simulink model "untitled"  (R2022b)
settings: Solver=VariableStepAuto  StartTime=0.0  StopTime=10.0  RelTol=1e-3
settings Model: Creator=Dell  LastModifiedBy=Dell

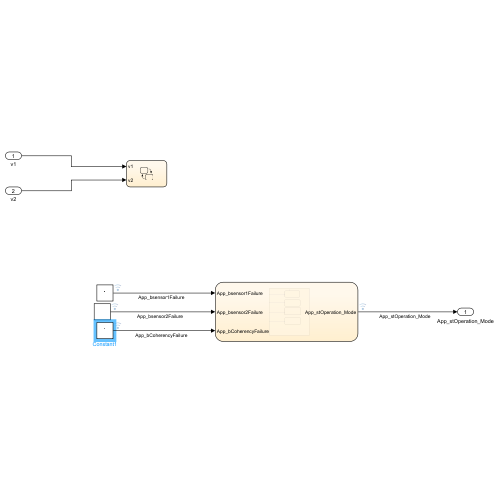
[thumbnail: Simulink's stored preview of the top-level diagram]
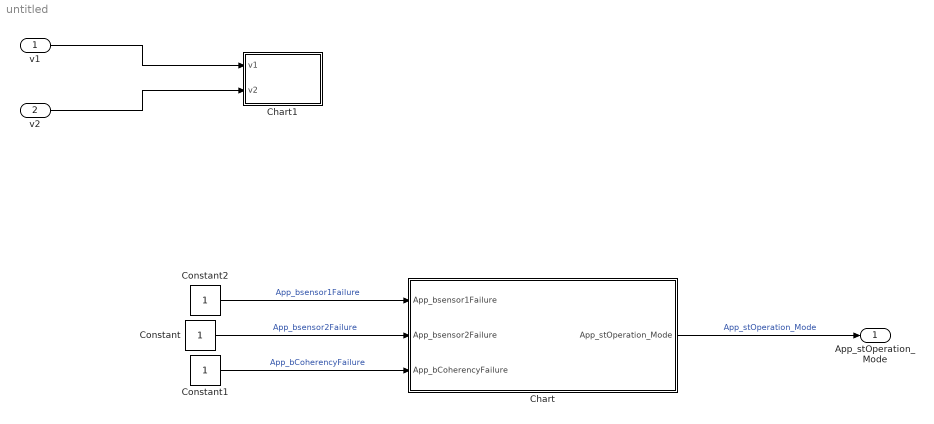
== system untitled ==
  v1 : Inport
  v2 : Inport  Port=2
  Chart : Stateflow chart  TreatAsAtomicUnit=on
  Chart1 : Stateflow chart  TreatAsAtomicUnit=on
      settings: PortSchema="{\"entries\":[{\"content\":{\"sides\":[{\"content\":{\"connectorIds\":[\"In2\",\"In1\"]},\"type\":\"ConnectorPlacement.EquallySpacedRectSide\",\"uuid\":\"969f0c33-844b-45d6-9c47-d424376eedef\"},{\"content\":{\"connectorIds\":[],\"side\":\"RIGHT\"},\"type\":\"ConnectorPlacement.EquallySpacedRectSide\",\"uuid\":\"6fc1ba59-4f2d-4ccb-a718-6a4f6694da1f\"},{\"content\":{\"connectorIds\":[],\"side\":\"TOP\"},\"type\":\"ConnectorPlacement.EquallySpacedRectSide\",\"uuid\":\"641840c5-dfaf-4b15-b882-b875e40945c1\"},{\"content\":{\"connectorIds\":[],\"side\":\"BOTTOM\"},\"type\":\"ConnectorPlacement.EquallySpacedRectSide\",\"uuid\":\"7f94b3d5-1be1-4166-8959-cf71582b0859\"}]},\"type\":\"ConnectorPlacement.EquallySpacedConnector\",\"uuid\":\"08648014-848e-4dc1-af57-bd70b5d3173f\"}],\"packageUris\":[\"http://schema.mathworks.com/mf0/Connector/R2020b\"],\"version\":\"1.0\"}"
  Constant : Constant
  Constant1 : Constant
  Constant2 : Constant
  App_stOperation_Mode : Outport  OutDataTypeStr=Enum: App_modes
  wires:
  Constant2/1 -> Chart/1(App_bsensor1Failure)  "App_bsensor1Failure"
  Constant/1 -> Chart/2(App_bsensor2Failure)  "App_bsensor2Failure"
  Constant1/1 -> Chart/3(App_bCoherencyFailure)  "App_bCoherencyFailure"
  Chart/1(App_stOperation_Mode) -> App_stOperation_Mode/1  "App_stOperation_Mode"
  v1/1 -> Chart1/2(v1)
  v2/1 -> Chart1/1(v2)

== stateflow chart untitled/Chart1 ==
  data: v2 input; v1 input

== stateflow chart untitled/Chart ==
  state Modes
    state Normal
      entry:
      App_stOperation_Mode=App_modes.Normal;
    state Downgraded_Sen1
      entry:
      App_stOperation_Mode=App_modes.Downgraded_sen_1;
    state Downgraded_Sen2
      entry:
      App_stOperation_Mode=App_modes.Downgraded_sen_2;
    state Failure
      entry:
      App_stOperation_Mode=App_modes.Failure;
    (default) -> Normal
    Modes -> Normal [order 1] : [~App_bCoherencyFailure && ~App_bsensor2Failure && ~App_bsensor1Failure]
    Modes -> Downgraded_Sen1 [order 3] : [[App_bsensor2Failure && ~App_bsensor1Failure]]
    Modes -> Downgraded_Sen2 [order 4] : [[~App_bsensor2Failure && App_bsensor1Failure]]
    Modes -> Failure [order 2] : [App_bCoherencyFailure]
  data: App_bsensor1Failure input; App_bsensor2Failure input; App_bCoherencyFailure input; App_stOperation_Mode output
